simulink model "path_tracking_error_calculation"  (R2025b)
settings: Solver=VariableStepAuto  StartTime=0.0  StopTime=10.0  RelTol=1e-3
values from neighbouring files (symbols this model uses):
  xRef = refPose(:,1)    [autoware_referance_path_creater.m]    (also in pure_pursuit_parameters.m)
  yRef = refPose(:,2)    [autoware_referance_path_creater.m]    (also in pure_pursuit_parameters.m)
settings Model: Creator=omer  LastModifiedBy=omer

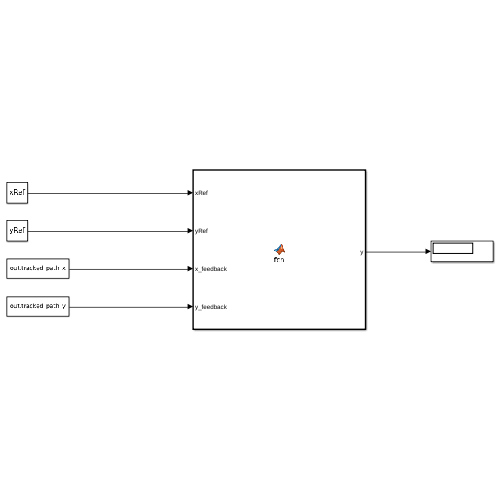
[thumbnail: Simulink's stored preview of the top-level diagram]
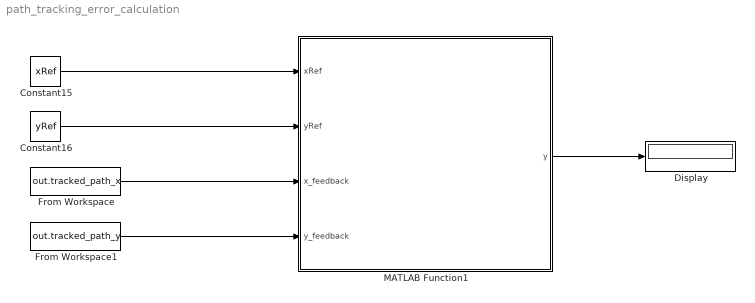
== system path_tracking_error_calculation ==
  Constant15 : Constant  Value=xRef
  Constant16 : Constant  Value=yRef
  Display : Display
  From Workspace : FromWorkspace  VariableName=out.tracked_path_x
  From Workspace1 : FromWorkspace  VariableName=out.tracked_path_y
  MATLAB Function1 : MATLAB Function  TreatAsAtomicUnit=on
  wires:
  From Workspace/1 -> MATLAB Function1/3(x_feedback)
  Constant15/1 -> MATLAB Function1/1(xRef)
  Constant16/1 -> MATLAB Function1/2(yRef)
  From Workspace1/1 -> MATLAB Function1/4(y_feedback)
  MATLAB Function1/1(y) -> Display/1

== matlab function path_tracking_error_calculation/MATLAB Function1 ==
  data: xRef input; y output; yRef input; x_feedback input; y_feedback input
function y = fcn(xRef, yRef, x_feedback, y_feedback)

        plot(xRef,yRef);
        hold on;
        plot(x_feedback,y_feedback);
        legend("ref","tracked path");
        y = 1;
